simulink model "test_qdr_vacc"  (Simulink 7.0)
settings: Solver=ode45  StartTime=0.0  StopTime=57000  RelTol=1e-3
undefined symbols (not defined in the file): Down, Up
libraries: xbsIndex_r4 x308, xps_library x14, casper_library x9, xbsReplacements_r4 x6
(part 3 of 3)

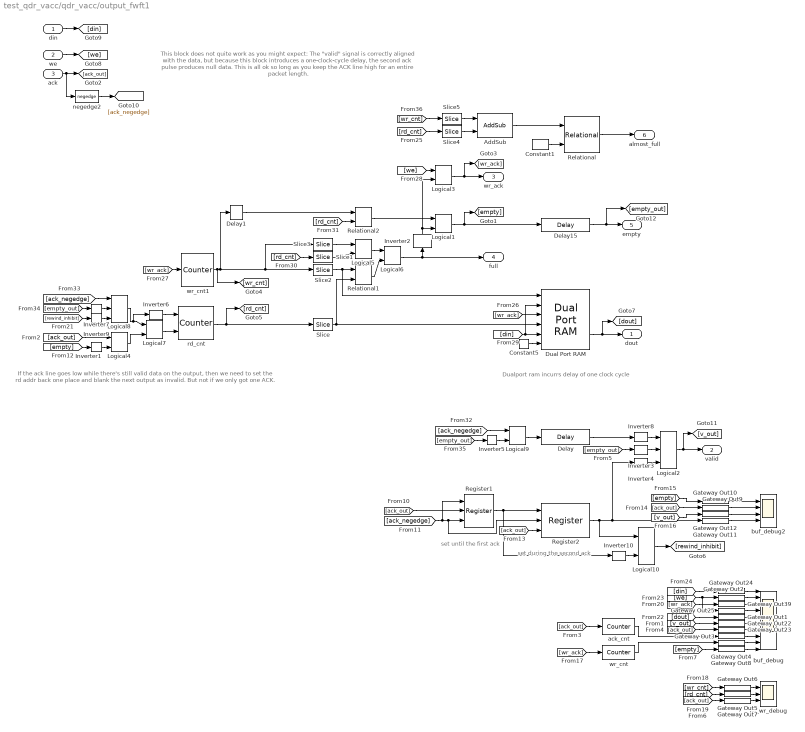
== system test_qdr_vacc/qdr_vacc/output_fwft1 ==
  note: Dualport ram incurrs delay
      | of one clock cycle
  note: If the ack line goes low while there's still valid data on the output,
      | then we need to set the rd addr back one place and blank the next
      | output as invalid. But not if we only got one ACK.
  note: set during the second ack
  note: set until the first ack
  note: This block does not quite work as you might expect:
      | The "valid" signal is correctly aligned with the data,
      | but because this block introduces a one-clock-cycle delay,
      | the second ack pulse produces null data.
      |
      | This is all ok so long as you keep the ACK line high for an entire packet length.
  din : Inport  OutDataType=sfix(16)  OutScaling=2^0
  we : Inport  Port=2  OutDataType=sfix(16)  OutScaling=2^0
  ack : Inport  Port=3  OutDataType=sfix(16)  OutScaling=2^0
  AddSub : xbsIndex_r4/AddSub  mode=Subtraction  use_carryin=off  use_carryout=off  en=off  latency=0  precision=User Defined  arith_type=Unsigned  n_bits=depth_bits  bin_pt=0  quantization=Truncate  overflow=Wrap  dbl_ovrd=off  use_behavioral_HDL=off  pipelined=on  use_rpm=on  hw_selection=Fabric  block_type=addsub
      settings: block_version=10.1.3
  Constant1 : xbsIndex_r4/Constant  arith_type=Unsigned  const=(2^depth_bits) - 2^(burst_bits)-1  n_bits=depth_bits+1  bin_pt=0  explicit_period=on  period=1  equ=P=C  opselect=C  inp2=PCIN>>17  opr=+  inp1=P  carry=CIN  dbl_ovrd=off  block_type=constant
  Constant5 : xbsIndex_r4/Constant  arith_type=Boolean  const=0  n_bits=1  bin_pt=0  explicit_period=on  period=1  equ=P=C  opselect=C  inp2=PCIN>>17  opr=+  inp1=P  carry=CIN  dbl_ovrd=off  block_type=constant
  Delay : xbsIndex_r4/Delay  en=off  latency=1  dbl_ovrd=off  reg_retiming=on  block_type=delay
      settings: xl_area=[0, 0, 0, 0, 0, 0, 0]
  Delay1 : xbsIndex_r4/Delay  en=off  latency=1  dbl_ovrd=off  reg_retiming=on  block_type=delay
  Delay15 : xbsIndex_r4/Delay  en=off  latency=1  dbl_ovrd=off  reg_retiming=on  block_type=delay
      settings: xl_area=[0, 0, 0, 0, 0, 0, 0]
  Dual Port RAM : xbsIndex_r4/Dual Port RAM  depth=2^depth_bits  initVector=0  distributed_mem=Block RAM  init_a=0  init_b=0  rst_a=off  rst_b=off  en_a=off  en_b=off  latency=1  write_mode_A=Read Before Write  write_mode_B=Read Before Write  dbl_ovrd=off  optimize=Area  use_rpm=off  block_type=dpram
      settings: xl_area=[0, 0, 0, 0, 0, 0, 0]  block_version=10.1.3
  Gateway Out{1..12,22..25,39} (17 alike) : xbsIndex_r4/Gateway Out  hdl_port=on  timing_constraint=None  locs_specified=off  LOCs={}  block_type=gatewayout
      settings: infoedit="Gateway out block.  Converts Xilinx fixed point inputs into ouputs of type Simulink integer, double, or fixed point.<P><P>Hardware notes:  In hardware these blocks become top level output ports or are discarded, depending on how they are configured."  xl_area=[0, 0, 0, 0, 0, 0, 0]  block_version=10.1.3
  Inverter{1,3..10} (9 alike) : xbsIndex_r4/Inverter  en=off  latency=0  dbl_ovrd=off  block_type=inv
      settings: xl_area=[0, 0, 0, 0, 0, 0, 0]
  Inverter2 : xbsIndex_r4/Inverter  Orientation=up  en=off  latency=0  dbl_ovrd=off  block_type=inv
      settings: xl_area=[0, 0, 0, 0, 0, 0, 0]
  Logical{1,3..4,6,9..10} (6 alike) : xbsIndex_r4/Logical  logical_function=AND  inputs=2  en=off  latency=0  precision=Full  arith_type=Unsigned  n_bits=8  bin_pt=2  align_bp=on  dbl_ovrd=off  block_type=logical
      settings: xl_area=[0, 0, 0, 0, 0, 0, 0]
  Logical2 : xbsIndex_r4/Logical  logical_function=AND  inputs=3  en=off  latency=0  precision=Full  arith_type=Unsigned  n_bits=8  bin_pt=2  align_bp=on  dbl_ovrd=off  block_type=logical
      settings: xl_area=[0, 0, 0, 0, 0, 0, 0]
  Logical5 : xbsIndex_r4/Logical  logical_function=XOR  inputs=2  en=off  latency=0  precision=Full  arith_type=Unsigned  n_bits=8  bin_pt=2  align_bp=on  dbl_ovrd=off  block_type=logical
      settings: xl_area=[0, 0, 0, 0, 0, 0, 0]
  Logical7 : xbsIndex_r4/Logical  logical_function=OR  inputs=2  en=off  latency=0  precision=Full  arith_type=Unsigned  n_bits=8  bin_pt=2  align_bp=on  dbl_ovrd=off  block_type=logical
      settings: xl_area=[0, 0, 0, 0, 0, 0, 0]
  Logical8 : xbsIndex_r4/Logical  logical_function=AND  inputs=3  en=off  latency=0  precision=Full  arith_type=Unsigned  n_bits=8  bin_pt=2  align_bp=on  dbl_ovrd=off  block_type=logical
      settings: xl_area=[0, 0, 0, 0, 0, 0, 0]
  Register1 : xbsIndex_r4/Register  init=0  rst=on  en=on  dbl_ovrd=off  block_type=register
      settings: xl_area=[0, 0, 0, 0, 0, 0, 0]
  Register2 : xbsIndex_r4/Register  init=0  rst=on  en=on  dbl_ovrd=off  block_type=register
      settings: xl_area=[0, 0, 0, 0, 0, 0, 0]
  Relational : xbsIndex_r4/Relational  mode=a>b  en=off  latency=1  dbl_ovrd=off  block_type=relational
      settings: block_version=10.1.3
  Relational1 : xbsIndex_r4/Relational  mode=a=b  en=off  latency=0  dbl_ovrd=off  block_type=relational
      settings: xl_area=[0, 0, 0, 0, 0, 0, 0]  block_version=10.1.3
  Relational2 : xbsIndex_r4/Relational  mode=a=b  en=off  latency=0  dbl_ovrd=off  block_type=relational
      settings: xl_area=[0, 0, 0, 0, 0, 0, 0]  block_version=10.1.3
  Slice{,2,4..5} (4 alike) : xbsIndex_r4/Slice  nbits=1  boolean_output=off  mode=Two Bit Locations  bit1=-1  base1=MSB of Input  bit0=0  base0=LSB of Input  dbl_ovrd=off  block_type=slice
      settings: infoedit="Extracts a given range of bits from each input sample and presents it at the output.  The output type is ordinarily unsigned with binary point at zero, but can be Boolean when the slice is one bit wide.<P><P>Hardware notes: In hardware this block costs nothing."  block_version=10.1.3
  Slice1 : xbsIndex_r4/Slice  nbits=1  boolean_output=on  mode=Upper Bit Location + Width  bit1=0  base1=MSB of Input  bit0=0  base0=LSB of Input  dbl_ovrd=off  block_type=slice
      settings: infoedit="Extracts a given range of bits from each input sample and presents it at the output.  The output type is ordinarily unsigned with binary point at zero, but can be Boolean when the slice is one bit wide.<P><P>Hardware notes: In hardware this block costs nothing."  block_version=10.1.3
  Slice3 : xbsIndex_r4/Slice  nbits=1  boolean_output=on  mode=Upper Bit Location + Width  bit1=0  base1=MSB of Input  bit0=0  base0=LSB of Input  dbl_ovrd=off  block_type=slice
      settings: infoedit="Extracts a given range of bits from each input sample and presents it at the output.  The output type is ordinarily unsigned with binary point at zero, but can be Boolean when the slice is one bit wide.<P><P>Hardware notes: In hardware this block costs nothing."  block_version=10.1.3
  ack_cnt : xbsIndex_r4/Counter  cnt_type=Free Running  cnt_to=Inf  operation=Up  start_count=0  cnt_by_val=1  arith_type=Unsigned  n_bits=depth_bits + 1  bin_pt=0  load_pin=off  rst=off  en=on  explicit_period=on  period=1  dbl_ovrd=off  use_behavioral_HDL=off  use_rpm=on  implementation=Fabric  block_type=counter
      settings: xl_area=[0, 0, 0, 0, 0, 0, 0]
  buf_debug : Scope  NumInputPorts=10
      settings: YMin=12000~0~9500~0~15500~-5~-5~-5~-5~-5  YMax=13300~1~10500~1~17250~5~5~5~5~5  SaveName=ScopeData13
  buf_debug2 : Scope  NumInputPorts=4
      settings: YMin=0~0.95~0~-1  YMax=1~1.05~1~1  SaveName=ScopeData15
  negedge2 : casper_library/Misc/negedge  Tag=Rising Edge Detector  SystemSampleTime=-1
  rd_cnt : xbsIndex_r4/Counter  cnt_type=Free Running  cnt_to=Inf  operation=Up/Down  start_count=0  cnt_by_val=1  arith_type=Unsigned  n_bits=depth_bits + 1  bin_pt=0  load_pin=off  rst=off  en=on  explicit_period=on  period=1  dbl_ovrd=off  use_behavioral_HDL=off  use_rpm=on  implementation=Fabric  block_type=counter
      settings: xl_area=[0, 0, 0, 0, 0, 0, 0]
  rd_wr_debug : Scope  NumInputPorts=3
      settings: YMin=150~0~0  YMax=300~1~1  SaveName=ScopeData14
  wr_cnt : xbsIndex_r4/Counter  cnt_type=Free Running  cnt_to=Inf  operation=Up  start_count=0  cnt_by_val=1  arith_type=Unsigned  n_bits=depth_bits + 1  bin_pt=0  load_pin=off  rst=off  en=on  explicit_period=on  period=1  dbl_ovrd=off  use_behavioral_HDL=off  use_rpm=on  implementation=Fabric  block_type=counter
      settings: xl_area=[0, 0, 0, 0, 0, 0, 0]
  wr_cnt1 : xbsIndex_r4/Counter  cnt_type=Free Running  cnt_to=Inf  operation=Up  start_count=0  cnt_by_val=1  arith_type=Unsigned  n_bits=depth_bits + 1  bin_pt=0  load_pin=off  rst=off  en=on  explicit_period=on  period=1  dbl_ovrd=off  use_behavioral_HDL=off  use_rpm=on  implementation=Fabric  block_type=counter
      settings: xl_area=[0, 0, 0, 0, 0, 0, 0]
  dout : Outport  OutDataType=sfix(16)  OutScaling=2^0
  valid : Outport  Port=2  OutDataType=sfix(16)  OutScaling=2^0
  wr_ack : Outport  Port=3  OutDataType=sfix(16)  OutScaling=2^0
  full : Outport  Port=4  OutDataType=sfix(16)  OutScaling=2^0
  empty : Outport  Port=5  OutDataType=sfix(16)  OutScaling=2^0
  almost_full : Outport  Port=6  OutDataType=sfix(16)  OutScaling=2^0
  wires:
  Delay1/1 -> Relational2/1
  [wr_ack] -> wr_cnt1/1
  Delay15/1 -> [empty_out], empty/1
  [empty_out] -> Inverter3/1
  Inverter8/1 -> Logical2/1
  Inverter4/1 -> Logical2/3
  Delay/1 -> Inverter8/1
  Logical9/1 -> Delay/1
  Inverter5/1 -> Logical9/2
  [empty_out] -> Inverter5/1
  [ack_negedge] -> Logical9/1
  Inverter7/1 -> Logical8/2
  [empty_out] -> Inverter7/1
  [ack_negedge] -> Logical8/1
  Logical8/1 -> Logical7/1, Inverter6/1
  Logical4/1 -> Logical7/2
  Logical7/1 -> rd_cnt/2
  Inverter6/1 -> rd_cnt/1
  negedge2/1 -> [ack_negedge]
  Register2/1 -> Inverter4/1, Gateway Out11/1, Logical10/1
  [rd_cnt] -> Relational2/2
  [rd_cnt] -> Slice1/1
  din/1 -> [din]
  [din] -> Dual Port RAM/5, Dual Port RAM/2
  Logical3/1 -> [wr_ack], wr_ack/1
  [we] -> Logical3/1
  [wr_ack] -> Dual Port RAM/3
  [din] -> Gateway Out24/1
  [we] -> Gateway Out25/1, Gateway Out2/1
  [dout] -> Gateway Out1/1
  [wr_ack] -> Gateway Out39/1
  [rd_cnt] -> Gateway Out5/1
  [wr_cnt] -> Gateway Out6/1
  [wr_ack] -> wr_cnt/1
  [ack_out] -> Register2/3
  [v_out] -> Gateway Out12/1
  [empty] -> Gateway Out10/1
  [ack_out] -> Gateway Out9/1
  Gateway Out11/1 -> buf_debug2/4
  Gateway Out12/1 -> buf_debug2/3
  Gateway Out9/1 -> buf_debug2/2
  Gateway Out10/1 -> buf_debug2/1
  Register1/1 -> Register2/1, Inverter10/1
  [ack_out] -> Register1/2
  [ack_negedge] -> Register2/2, Register1/3, Register1/1
  Logical2/1 -> [v_out], valid/1
  Inverter1/1 -> Logical4/2
  [empty] -> Gateway Out8/1
  Gateway Out8/1 -> buf_debug/10
  [ack_out] -> Gateway Out7/1
  Gateway Out7/1 -> rd_wr_debug/3
  Gateway Out5/1 -> rd_wr_debug/2
  Gateway Out6/1 -> rd_wr_debug/1
  [ack_out] -> Gateway Out23/1
  [ack_out] -> ack_cnt/1
  [ack_out] -> Logical4/1
  ack/1 -> negedge2/1, [ack_out]
  [v_out] -> Gateway Out22/1
  [empty] -> Inverter1/1
  wr_cnt/1 -> Gateway Out4/1
  ack_cnt/1 -> Gateway Out3/1
  Gateway Out4/1 -> buf_debug/9
  Gateway Out3/1 -> buf_debug/8
  Gateway Out23/1 -> buf_debug/7
  Gateway Out22/1 -> buf_debug/6
  Gateway Out1/1 -> buf_debug/5
  Gateway Out25/1 -> buf_debug/4
  Gateway Out39/1 -> buf_debug/3
  Gateway Out2/1 -> buf_debug/2
  Gateway Out24/1 -> buf_debug/1
  Logical1/1 -> Delay15/1, [empty]
  Dual Port RAM/2 -> [dout], dout/1
  Constant5/1 -> Dual Port RAM/6
  we/1 -> [we]
  Inverter2/1 -> Logical3/2, Logical1/2
  rd_cnt/1 -> Slice/1, [rd_cnt]
  wr_cnt1/1 -> Delay1/1, Slice2/1, Slice3/1, [wr_cnt]
  Slice/1 -> Dual Port RAM/4, Relational1/2
  Slice2/1 -> Dual Port RAM/1, Relational1/1
  Slice3/1 -> Logical5/1
  Slice1/1 -> Logical5/2
  Relational1/1 -> Logical6/2
  Logical5/1 -> Logical6/1
  Logical6/1 -> full/1, Inverter2/1
  Relational2/1 -> Logical1/1
  [rd_cnt] -> Slice4/1
  [wr_cnt] -> Slice5/1
  AddSub/1 -> Relational/1
  Relational/1 -> almost_full/1
  Constant1/1 -> Relational/2
  Slice5/1 -> AddSub/1
  Slice4/1 -> AddSub/2
  Inverter9/1 -> Logical8/3
  [rewind_inhibit] -> Inverter9/1
  Inverter10/1 -> Logical10/2
  Logical10/1 -> [rewind_inhibit]
  Inverter3/1 -> Logical2/2

== system test_qdr_vacc/qdr_vacc/acc_ctrl/pulse_ext ==
  in : Inport  OutDataType=sfix(16)  OutScaling=2^0
  Constant5 : xbsIndex_r4/Constant  arith_type=Unsigned  const=pulse_len  n_bits=bits  bin_pt=0  explicit_period=off  period=1  equ=P=C  opselect=C  inp2=PCIN>>17  opr=+  inp1=P  carry=CIN  dbl_ovrd=off  block_type=constant
      settings: block_version=9.1.01
  Counter3 : xbsIndex_r4/Counter  cnt_type=Free Running  cnt_to=1023  operation=Up  start_count=0  cnt_by_val=1  arith_type=Unsigned  n_bits=bits  bin_pt=0  load_pin=off  rst=on  en=on  explicit_period=on  period=1  dbl_ovrd=off  use_behavioral_HDL=off  use_rpm=on  implementation=Fabric  block_type=counter
      settings: xl_area=[0, 0, 0, 0, 0, 0, 0]  block_version=9.1.01
  Logical : xbsIndex_r4/Logical  logical_function=AND  inputs=2  en=off  latency=0  precision=Full  arith_type=Unsigned  n_bits=16  bin_pt=0  align_bp=on  dbl_ovrd=off  block_type=logical
  Logical1 : xbsIndex_r4/Logical  logical_function=OR  inputs=2  en=off  latency=0  precision=Full  arith_type=Unsigned  n_bits=16  bin_pt=0  align_bp=on  dbl_ovrd=off  block_type=logical
  Register : xbsIndex_r4/Register  init=0  rst=off  en=on  dbl_ovrd=off  block_type=register
  Relational5 : xbsIndex_r4/Relational  mode=a!=b  en=off  latency=0  dbl_ovrd=off  block_type=relational
      settings: xl_area=[0, 0, 0, 0, 0, 0, 0]  block_version=9.1.01
  out : Outport  OutDataType=sfix(16)  OutScaling=2^0
  wires:
  in/1 -> Register/1, Register/2, Counter3/1, Logical1/1
  Relational5/1 -> Counter3/2, Logical/1
  Constant5/1 -> Relational5/2
  Counter3/1 -> Relational5/1
  Register/1 -> Logical/2
  Logical/1 -> Logical1/2
  Logical1/1 -> out/1
